simulink model "MotGenEvDynamic"  (R2022b)
settings: Solver=ode1  StartTime=0.0  StopTime=inf  FixedStep=TsElecDrive  RelTol=1e-3  EnableMultiTasking=on
model workspace (MAT data in the model file):
  EV_current = 200
  EV_motion = [20 4 0.8]
  EV_sf = 2000
  Fs = 0
  Fv = 0.0025
  Jcomp = 0.0227
  Ki = 25.1327
  Kisa = 346.6583
  Kp_d = 0.077049
  Kp_q = 0.1541
  Ksa = 85.4316
  Ksf = 1996.2651
  Ld = 6.13138564528e-05
  Ldq = [0.00075852 0.00084286]
  Lq = 0.000122627712906
  Mechanical = [0.0227 0.0025 0]
  P = 4
  PolePairs = 4
  Rs = 0.02
  T_max = 450
  T_mtpa = [0 42.1986572825 85.2083176897 129.729081531 176.299639273 225.306651971 277.019503371 331.625177598 389.25482581 450.002001304]
  ba = 3.4029
  id_mtpa = [0 -7.80314458768 -30.092823648 -64.186681647 -107.097717515 -156.321290228 -210.017144052 -266.906008079 -326.111998186 -387.032483343]
  idq0 = [0 0]
  idq_limits = [-387.027355555 779.385063397 870.190353311]
  iq_mtpa = [0 96.3724280977 191.019783835 282.872542968 371.626993516 457.46803527 540.777238675 621.964104296 701.396562769 779.382517017]
  lambda_pm = 0.0725
  mechanical = [0.0227 0.0025 0]
  omega_init = 0
  theta_init = 0
undefined symbols (not defined in the file): IO334, J, T_cpu, Tcpu, TsEV
libraries: speedgoatlib_hdlCoder_IO3xx x24, autolibmotorctrlr x1, HDL_Motor_Lib x1
settings Model: ModifiedByFormat=The MathWorks, Inc.  PauseTimes=10  Creator=The MathWorks, Inc.  LastModifiedBy=The MathWorks, Inc.
settings SolverCC: ConcurrentTasks=on  AlgebraicLoopSolver=TrustRegion  PositivePriorityOrder=on  AutoInsertRateTranBlk=on  DecoupledContinuousIntegration=on  MaxZcPerStep=1
settings DataIOCC: DSMLogging=off  ReturnWorkspaceOutputs=off
settings OptimizationCC: BlockReduction=off  UseFloatMulNetSlope=on  OptimizeBlockIOStorage=off
settings DebuggingCC: UnderspecifiedInitializationDetection=Classic  MergeDetectMultiDrivingBlocksExec=none  TasksWithSamePriorityMsg=none  UnconnectedInputMsg=warning  UnconnectedOutputMsg=warning  UnconnectedLineMsg=warning  SFMachineParentedDataDiag=warning  ArithmeticOperatorsInVariantConditions=warning
settings HardwareCC: ProdBitPerLong=64  ProdLongLongMode=on  ProdHWDeviceType=Intel->x86-64 (Linux 64)
settings ModelReferenceCC: EnableRefExpFcnMdlSchedulingChecks=on  PropagateSignalLabelsOutOfModel=off
settings SFSimCC: SimUseLocalCustomCode=off  MATLABDynamicMemAlloc=off  CustomCodeUndefinedFunction=UseInterfaceOnly
settings RTWCC: Description=Simulink Real-Time  SystemTargetFile=slrealtime.tlc  TemplateMakefile=slrealtime_default_tmf  RTWUseLocalCustomCode=off  Toolchain=Simulink Real-Time Toolchain  BuildConfiguration=Faster Runs  CodeExecutionProfiling=on  TargetLang=C++  DLArmComputeVersion=19.05
settings CodeAppCC: StateflowObjectComments=on
settings ConfigComp: CovMetricSettings=dsw  CovSaveCumulativeToWorkspaceVar=on  CovSaveSingleToWorkspaceVar=on  CovExternalEMLEnable=off
settings SimscapeCC: SimscapeNormalizeSystem=off

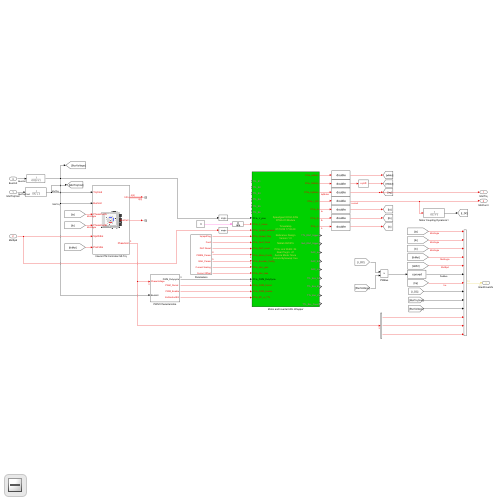
[thumbnail: Simulink's stored preview of the top-level diagram]
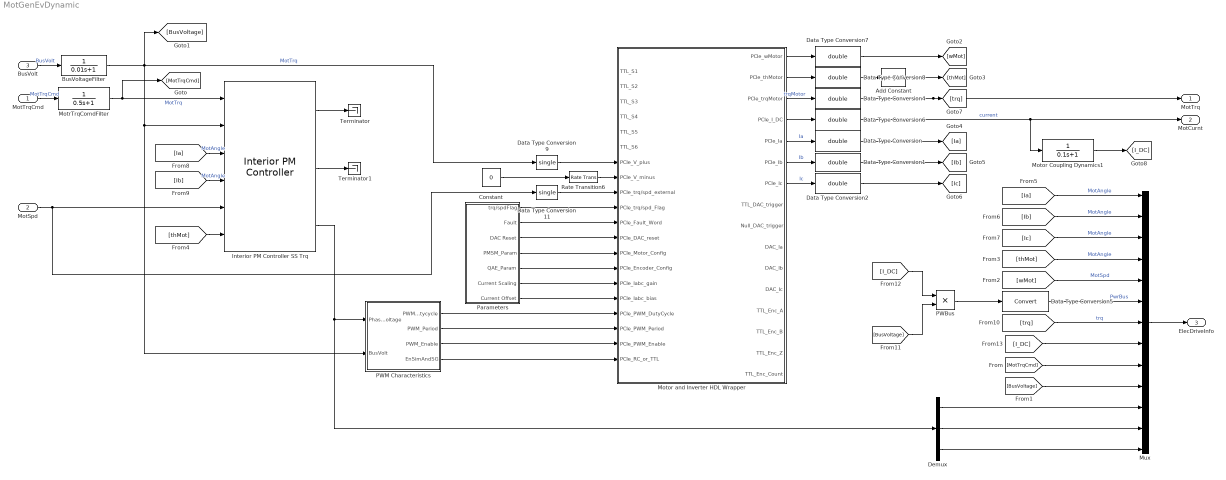
== system MotGenEvDynamic ==
  MotTrqCmd : Inport  OutDataTypeStr=double
  MotSpd : Inport  Port=2  OutDataTypeStr=double
  BusVolt : Inport  Port=3  OutDataTypeStr=double
  Add Constant : Bias  Bias=-pi/8  SaturateOnIntegerOverflow=off
  BusVoltageFilter : TransferFcn  Denominator=[0.01 1]
  Constant : Constant  Value=0  OutDataTypeStr=single
  Data Type Conversion{,1..2,4,6..8} (7 alike) : DataTypeConversion  OutDataTypeStr=double  SaturateOnIntegerOverflow=off  RndMeth=Floor
  Data Type Conversion11 : DataTypeConversion  OutDataTypeStr=single  SaturateOnIntegerOverflow=off  RndMeth=Floor
  Data Type Conversion5 : DataTypeConversion  SaturateOnIntegerOverflow=off  RndMeth=Floor
  Data Type Conversion9 : DataTypeConversion  OutDataTypeStr=single  SaturateOnIntegerOverflow=off  RndMeth=Floor
  Demux : Demux  Outputs=3
  Interior PM Controller SS Trq : autolibmotorctrlr/Interior PM Controller  control_type=Torque Control  Rs=Rs  Ld=Ld  Lq=Lq  lambda_pm=lambda_pm  PolePairs=PolePairs  Mechanical=Mechanical  MotorConstraint=Maximum Torque  T_max=T_max  I_max=44  bp=10  T_mtpa=T_mtpa  id_mtpa=id_mtpa  iq_mtpa=iq_mtpa  idq_limits=idq_limits  EV_current=EV_current  Tst=TsElecDrive  Kp_d=Kp_d  Kp_q=Kp_q  Ki=Ki/10  EV_motion=EV_motion  EV_sf=EV_sf  ba=ba  Ksa=Ksa  Kisa=Kisa  Ksf=Ksf  Jcomp=Jcomp  Fv=Fv  Fs=Fs  param_loss=Single efficiency measurement  eff=98  w_loss_bp=[0 200 400 600 800 1000]  T_loss_bp=[0 25 50 75 100]  losses_table=[100 100 100 100 100;100 150 200 250 300;100 200 300 400 500;100 250 400 550 700;100 300 500 700 900;100 350 600 850 1100]  w_eff_bp=[200 400 600 800 1000]  T_eff_bp=[25 50 75 100]  efficiency_table=[96.2 98.1 98.7 99;98.1 99 99.4 99.5;98.7 99.4 99.6 99.7;99 99.5 99.7 99.8;99.2 99.6 99.7 99.8]  x_w_bp=[-1000 -800 -600 -400 -200 200 400 600 800 1000]  x_T_bp=[-100 -75 -50 -25 25 50 75 100]  x_losses_mat=[200.400801603196 225.67703109328 200.803212851408 201.612903225806 199.999999999997 200 225 200;160.320641282556 180.541624874624 201.005025125625 202.020202020203 200 200 180 160;180.541624874624 180.722891566267 181.086519114686 197.568389057748 194.999999999999 179.999999999997 180 180;201.005025125625 181.086519114686 202.020202020203 193.67991845056 190 200 179.999999999997 200;202.020202020203 197.568389057748 193.67991845056 197.505197505197 190 190 194.999999999999 200;200 194.999999999999 190 190 197.505197505197 193.67991845056 197.568389057748 202.020202020203;200 179.999999999997 200 190 193.67991845056 202.020202020203 181.086519114686 201.005025125625;180 180 179.999999999997 194.999999999999 197.568389057748 181.086519114686 180.722891566267 180.541624874624;160 180 200 200 202.020202020203 201.005025125625 180.541624874624 160.320641282556;200 225 200 199.999999999997 201.612903225806 200.803212851408 225.67703109328 200.400801603196]  Tsm=5e-4
  Motor Coupling Dynamics1 : TransferFcn  Denominator=[0.1 1]
  Motor and Inverter HDL Wrapper : Subsystem  mask(Speedgoat IO334-325k Interface Block){module_id=1, slot=-1, ts=TsEV, OutputRange=Auto (same as ADC), PullRPort0=pull-down, VioPort0=3.3V, PullRPort1=pull-down, VioPort1=3.3V, PullRPort2=pull-down, VioPort2=3.3V, PullRPort3=pull-down, VioPort3=3.3V, PullRPort4=pull-down, VioPort4=3.3V, PullRPort5=pull-down, VioPort5=3.3V, PullRPort6=pull-down, VioPort6=3.3V, FpgaFreq=200}
      mask prompts: module_id "FPGA Module Identifier:"; slot "PCI slot (-1: autosearch):"; ts "Sample time:"; OutputRange "DAC Voltage Range:"; PullRPort0 "pull resistor"; VioPort0 "I/O voltage"; PullRPort1 "pull resistor"; VioPort1 "I/O voltage"; PullRPort2 "pull resistor"; VioPort2 "I/O voltage"; PullRPort3 "pull resistor"; VioPort3 "I/O voltage"; PullRPort4 "pull resistor"; VioPort4 "I/O voltage"; PullRPort5 "pull resistor"; VioPort5 "I/O voltage"; PullRPort6 "pull resistor"; VioPort6 "I/O voltage"; FpgaFreq "FPGA Frequency [MHz]"
      mask help: Simulink Real-Time Interface Block for Speedgoat IO334-325k.
      mask init:
      | hdlslrt.backend.mfpgaparameters;
      mask Help: eval('speedgoatdoc_hdlc')
      mask TypeOptions OutputRange: IO334 DAC Setup/OutputRange
      mask TypeOptions PullRPort0: Port Settings -2x/PullRPort0
      mask Callback PullRPort0: sg_fpga_HDLCoder_io3xx_2x_m(2)
      mask TypeOptions VioPort0: Port Settings -2x/VioPort0
      mask Callback VioPort0: sg_fpga_HDLCoder_io3xx_2x_m(2)
      mask TypeOptions PullRPort1: Port Settings -2x/PullRPort1
      mask Callback PullRPort1: sg_fpga_HDLCoder_io3xx_2x_m(2)
      mask TypeOptions VioPort1: Port Settings -2x/VioPort1
      mask Callback VioPort1: sg_fpga_HDLCoder_io3xx_2x_m(2)
      mask TypeOptions PullRPort2: Port Settings -2x/PullRPort2
      mask Callback PullRPort2: sg_fpga_HDLCoder_io3xx_2x_m(2)
      mask TypeOptions VioPort2: Port Settings -2x/VioPort2
      mask Callback VioPort2: sg_fpga_HDLCoder_io3xx_2x_m(2)
      mask TypeOptions PullRPort3: Port Settings -2x/PullRPort3
      mask Callback PullRPort3: sg_fpga_HDLCoder_io3xx_2x_m(2)
      mask TypeOptions VioPort3: Port Settings -2x/VioPort3
      mask Callback VioPort3: sg_fpga_HDLCoder_io3xx_2x_m(2)
      mask TypeOptions PullRPort4: Port Settings -2x/PullRPort4
      mask Callback PullRPort4: sg_fpga_HDLCoder_io3xx_2x_m(2)
      mask TypeOptions VioPort4: Port Settings -2x/VioPort4
      mask Callback VioPort4: sg_fpga_HDLCoder_io3xx_2x_m(2)
      mask TypeOptions PullRPort5: Port Settings -2x/PullRPort5
      mask Callback PullRPort5: sg_fpga_HDLCoder_io3xx_2x_m(2)
      mask TypeOptions VioPort5: Port Settings -2x/VioPort5
      mask Callback VioPort5: sg_fpga_HDLCoder_io3xx_2x_m(2)
      mask TypeOptions PullRPort6: Port Settings -2x/PullRPort6
      mask Callback PullRPort6: sg_fpga_HDLCoder_io3xx_2x_m(2)
      mask TypeOptions VioPort6: Port Settings -2x/VioPort6
      mask Callback VioPort6: sg_fpga_HDLCoder_io3xx_2x_m(2)
      mask DialogControl AnalogOutput Prompt: Analog Output
      mask DialogControl IO33421 Prompt: IO334-21
      mask DialogControl port1 Prompt: Port 1
      mask DialogControl port2 Prompt: Port 2
      mask DialogControl port3 Prompt: Port 3
      mask DialogControl port4 Prompt: Port 4
      mask DialogControl port5 Prompt: Port 5
      mask DialogControl port6 Prompt: Port 6
      mask DialogControl port7 Prompt: Port 7
      mask Display:
      | SetupBlkPath = find_system(gcb, 'LookUnderMasks', 'all', 'FollowLinks', 'on', 'regexp', 'on', 'Name', 'IO3(\d|x){2}\s+Setup' );
      | SetupBlkPath = SetupBlkPath{1};
      | TS = get_param(SetupBlkPath,'timestamp_mcs');
      | disp(sprintf('Speedgoat IO334-325k\nFPGA I/O Module\n\nTimestamp\n%s\n\nReference Design\nVersion 1.0\n\nMatlab R2021b\n\nPCIe Link Width: X4\nRear Plugin: -21\nAurora Mode: None\nAurora Byteswap: true\n', TS))
  MotrTrqComdFilter : TransferFcn  Denominator=[0.5 1]
  Mux : Mux  Inputs=13
  PWBus : Product
  PWM Characteristics : Subsystem
  Parameters : Subsystem
  Rate Transition6 : RateTransition
  Terminator : Terminator
  Terminator1 : Terminator
  MotTrq : Outport  VectorParamsAs1DForOutWhenUnconnected=off
  MotCurnt : Outport  Port=2  VectorParamsAs1DForOutWhenUnconnected=off
  ElecDriveInfo : Outport  Port=3  OutDataTypeStr=double  VectorParamsAs1DForOutWhenUnconnected=off
  wires:
  BusVolt/1 -> BusVoltageFilter/1  "BusVolt"
  MotSpd/1 -> Interior PM Controller SS Trq/5, Data Type Conversion11/1
  Interior PM Controller SS Trq/2 -> Terminator1/1
  Interior PM Controller SS Trq/1 -> Terminator/1
  Mux/1 -> ElecDriveInfo/1
  Demux/1 -> Mux/11
  Demux/2 -> Mux/12
  Demux/3 -> Mux/13
  Constant/1 -> Rate Transition6/1
  Parameters/7(Current Offset) -> Motor and Inverter HDL Wrapper/16(PCIe_Iabc_bias)
  Motor and Inverter HDL Wrapper/3(PCIe_trqMotor) -> Data Type Conversion4/1  "trqMotor"
  Motor and Inverter HDL Wrapper/2(PCIe_thMotor) -> Data Type Conversion8/1
  Motor and Inverter HDL Wrapper/4(PCIe_I_DC) -> Data Type Conversion6/1
  MotTrqCmd/1 -> MotrTrqComdFilter/1  "MotTrqCmd"
  PWBus/1 -> Data Type Conversion5/1
  Parameters/1(trq/spdFlag) -> Motor and Inverter HDL Wrapper/10(PCIe_trq/spd_Flag)
  Data Type Conversion11/1 -> Motor and Inverter HDL Wrapper/9(PCIe_trq/spd_external)
  Rate Transition6/1 -> Motor and Inverter HDL Wrapper/8(PCIe_V_minus)
  Parameters/4(PMSM_Param) -> Motor and Inverter HDL Wrapper/13(PCIe_Motor_Config)
  Parameters/5(QAE_Param) -> Motor and Inverter HDL Wrapper/14(PCIe_Encoder_Config)
  [trq] -> Mux/7  "trq"
  Data Type Conversion5/1 -> Mux/6  "PwrBus"
  Motor and Inverter HDL Wrapper/5(PCIe_Ia) -> Data Type Conversion/1  "Ia"
  Motor and Inverter HDL Wrapper/6(PCIe_Ib) -> Data Type Conversion1/1  "Ib"
  Motor and Inverter HDL Wrapper/7(PCIe_Ic) -> Data Type Conversion2/1  "Ic"
  Data Type Conversion9/1 -> Motor and Inverter HDL Wrapper/7(PCIe_V_plus)
  PWM Characteristics/4(EnSimAndSG) -> Motor and Inverter HDL Wrapper/20(PCIe_RC_or_TTL)
  Data Type Conversion4/1 -> [trq], MotTrq/1
  Parameters/2(Fault) -> Motor and Inverter HDL Wrapper/11(PCIe_Fault_Word)
  [wMot] -> Mux/5  "MotSpd"
  Interior PM Controller SS Trq/3 -> PWM Characteristics/1(PhaseVoltage), Demux/1
  [MotTrqCmd] -> Mux/9
  [BusVoltage] -> Mux/10
  PWM Characteristics/1(PWM_Dutycycle) -> Motor and Inverter HDL Wrapper/17(PCIe_PWM_DutyCycle)
  PWM Characteristics/2("PWM_Period ") -> Motor and Inverter HDL Wrapper/18(PCIe_PWM_Period)
  PWM Characteristics/3(PWM_Enable) -> Motor and Inverter HDL Wrapper/19(PCIe_PWM_Enable)
  Parameters/3(DAC Reset) -> Motor and Inverter HDL Wrapper/12(PCIe_DAC_reset)
  Motor and Inverter HDL Wrapper/1(PCIe_wMotor) -> Data Type Conversion7/1
  Data Type Conversion7/1 -> [wMot]
  Add Constant/1 -> [thMot]
  [thMot] -> Mux/4  "MotAngle"
  Data Type Conversion8/1 -> Add Constant/1
  [thMot] -> Interior PM Controller SS Trq/6
  Data Type Conversion/1 -> [Ia]
  Data Type Conversion1/1 -> [Ib]
  Data Type Conversion2/1 -> [Ic]
  [Ib] -> Mux/2  "MotAngle"
  [Ia] -> Mux/1  "MotAngle"
  [Ic] -> Mux/3  "MotAngle"
  [Ia] -> Interior PM Controller SS Trq/3  "MotAngle"
  [Ib] -> Interior PM Controller SS Trq/4  "MotAngle"
  Data Type Conversion6/1 -> Motor Coupling Dynamics1/1, MotCurnt/1  "current"
  [BusVoltage] -> PWBus/2
  Motor Coupling Dynamics1/1 -> [I_DC]
  [I_DC] -> PWBus/1
  [I_DC] -> Mux/8
  Parameters/6(Current Scaling) -> Motor and Inverter HDL Wrapper/15(PCIe_Iabc_gain)
  MotrTrqComdFilter/1 -> Interior PM Controller SS Trq/1, [MotTrqCmd]  "MotTrq"
  BusVoltageFilter/1 -> PWM Characteristics/2(BusVolt), Interior PM Controller SS Trq/2, [BusVoltage], Data Type Conversion9/1  "MotTrq"

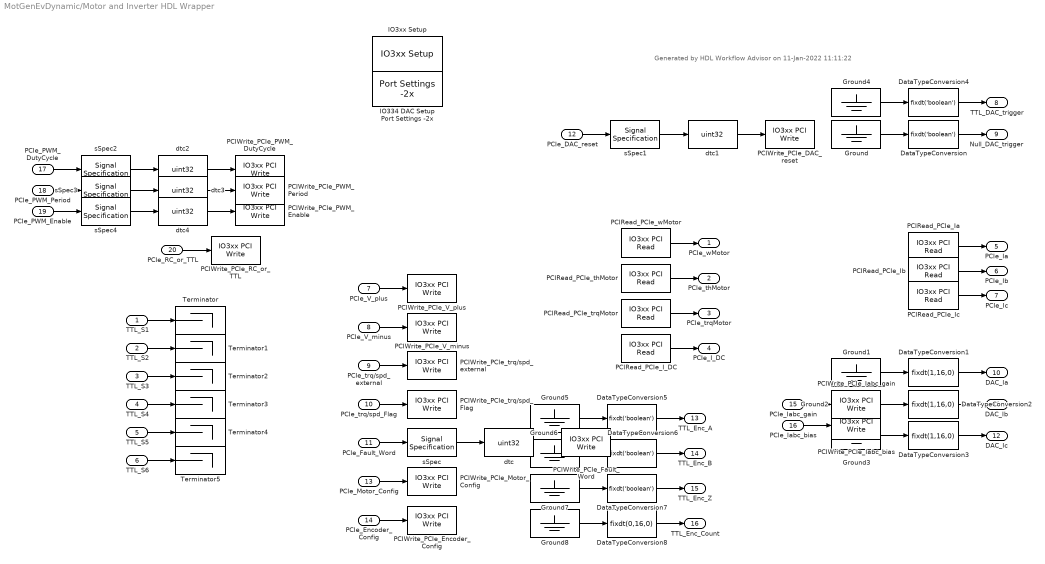
== system MotGenEvDynamic/Motor and Inverter HDL Wrapper ==
  note: Generated by HDL Workflow Advisor on 11-Jan-2022 11:11:22
  TTL_S1 : Inport
  TTL_S2 : Inport  Port=2
  TTL_S3 : Inport  Port=3
  TTL_S4 : Inport  Port=4
  TTL_S5 : Inport  Port=5
  TTL_S6 : Inport  Port=6
  PCIe_V_plus : Inport  Port=7
  PCIe_V_minus : Inport  Port=8
  PCIe_trq/spd_external : Inport  Port=9
  PCIe_trq/spd_Flag : Inport  Port=10
  PCIe_Fault_Word : Inport  Port=11
  PCIe_DAC_reset : Inport  Port=12
  PCIe_Motor_Config : Inport  Port=13
  PCIe_Encoder_Config : Inport  Port=14
  PCIe_Iabc_gain : Inport  Port=15
  PCIe_Iabc_bias : Inport  Port=16
  PCIe_PWM_DutyCycle : Inport  Port=17
  PCIe_PWM_Period : Inport  Port=18
  PCIe_PWM_Enable : Inport  Port=19
  PCIe_RC_or_TTL : Inport  Port=20
  DataTypeConversion{,4..7} (5 alike) : DataTypeConversion  OutDataTypeStr=fixdt('boolean')  ConvertRealWorld=Stored Integer (SI)  SaturateOnIntegerOverflow=off  RndMeth=Floor
  DataTypeConversion1 : DataTypeConversion  OutDataTypeStr=fixdt(1,16,0)  ConvertRealWorld=Stored Integer (SI)  SaturateOnIntegerOverflow=off  RndMeth=Floor
  DataTypeConversion2 : DataTypeConversion  OutDataTypeStr=fixdt(1,16,0)  ConvertRealWorld=Stored Integer (SI)  SaturateOnIntegerOverflow=off  RndMeth=Floor
  DataTypeConversion3 : DataTypeConversion  OutDataTypeStr=fixdt(1,16,0)  ConvertRealWorld=Stored Integer (SI)  SaturateOnIntegerOverflow=off  RndMeth=Floor
  DataTypeConversion8 : DataTypeConversion  OutDataTypeStr=fixdt(0,16,0)  ConvertRealWorld=Stored Integer (SI)  SaturateOnIntegerOverflow=off  RndMeth=Floor
  Ground{,1..8} (9 alike) : Ground
  IO334 DAC Setup : speedgoatlib_hdlCoder_IO3xx/IO334 DAC Setup  module_id=module_id  OutputRange=Auto (same as ADC)
  IO3xx Setup : speedgoatlib_hdlCoder_IO3xx/IO3xx Setup  mdl_ss_name=slrt_ex_pmsm/Motor and Inverter HDL Wrapper  board_type=IO334-325k  fpga_sync_mode=on  reset_mode=on  reset_mode_stop=off  device_id=1  module_id=module_id  pci_slot=slot  fpga_mat_file=hdl_prj\hdlsrc\slrt_ex_pmsm\MotorAndInverterHDLWrapper.mat  timestamp_mcs=01/10/22 17:02:49  timestamp=2201101544  tsreg=hex2dec('8')  bsf_file=MotorAndInverterHDLWrapperOriginal.mcs  mcs=0  init_reg_list=[]
  PCIRead_PCIe_I_DC : speedgoatlib_hdlCoder_IO3xx/IO3xx PCI Read  device_id=1  module_id=module_id  board_type=IO334-325k  port_name=PCIe_I_DC  port_offset=hex2dec('15C')  port_type=single  port_dim=1  strobe=0  sample_time=ts
  PCIRead_PCIe_Ia : speedgoatlib_hdlCoder_IO3xx/IO3xx PCI Read  device_id=1  module_id=module_id  board_type=IO334-325k  port_name=PCIe_Ia  port_offset=hex2dec('184')  port_type=single  port_dim=1  strobe=0  sample_time=ts
  PCIRead_PCIe_Ib : speedgoatlib_hdlCoder_IO3xx/IO3xx PCI Read  device_id=1  module_id=module_id  board_type=IO334-325k  port_name=PCIe_Ib  port_offset=hex2dec('188')  port_type=single  port_dim=1  strobe=0  sample_time=ts
  PCIRead_PCIe_Ic : speedgoatlib_hdlCoder_IO3xx/IO3xx PCI Read  device_id=1  module_id=module_id  board_type=IO334-325k  port_name=PCIe_Ic  port_offset=hex2dec('18C')  port_type=single  port_dim=1  strobe=0  sample_time=ts
  PCIRead_PCIe_thMotor : speedgoatlib_hdlCoder_IO3xx/IO3xx PCI Read  device_id=1  module_id=module_id  board_type=IO334-325k  port_name=PCIe_thMotor  port_offset=hex2dec('154')  port_type=single  port_dim=1  strobe=0  sample_time=ts
  PCIRead_PCIe_trqMotor : speedgoatlib_hdlCoder_IO3xx/IO3xx PCI Read  device_id=1  module_id=module_id  board_type=IO334-325k  port_name=PCIe_trqMotor  port_offset=hex2dec('158')  port_type=single  port_dim=1  strobe=0  sample_time=ts
  PCIRead_PCIe_wMotor : speedgoatlib_hdlCoder_IO3xx/IO3xx PCI Read  device_id=1  module_id=module_id  board_type=IO334-325k  port_name=PCIe_wMotor  port_offset=hex2dec('150')  port_type=single  port_dim=1  strobe=0  sample_time=ts
  PCIWrite_PCIe_DAC_reset : speedgoatlib_hdlCoder_IO3xx/IO3xx PCI Write  device_id=1  module_id=module_id  board_type=IO334-325k  port_name=PCIe_DAC_reset  port_offset=hex2dec('114')  port_type=uint32  port_dim=1  strobe=0  sample_time=ts
  PCIWrite_PCIe_Encoder_Config : speedgoatlib_hdlCoder_IO3xx/IO3xx PCI Write  device_id=1  module_id=module_id  board_type=IO334-325k  port_name=PCIe_Encoder_Config  port_offset=hex2dec('160')  port_type=single  port_dim=5  strobe=hex2dec('180')  sample_time=ts
  PCIWrite_PCIe_Fault_Word : speedgoatlib_hdlCoder_IO3xx/IO3xx PCI Write  device_id=1  module_id=module_id  board_type=IO334-325k  port_name=PCIe_Fault_Word  port_offset=hex2dec('110')  port_type=uint32  port_dim=1  strobe=0  sample_time=ts
  PCIWrite_PCIe_Iabc_bias : speedgoatlib_hdlCoder_IO3xx/IO3xx PCI Write  device_id=1  module_id=module_id  board_type=IO334-325k  port_name=PCIe_Iabc_bias  port_offset=hex2dec('11C')  port_type=single  port_dim=1  strobe=0  sample_time=ts
  PCIWrite_PCIe_Iabc_gain : speedgoatlib_hdlCoder_IO3xx/IO3xx PCI Write  device_id=1  module_id=module_id  board_type=IO334-325k  port_name=PCIe_Iabc_gain  port_offset=hex2dec('118')  port_type=single  port_dim=1  strobe=0  sample_time=ts
  PCIWrite_PCIe_Motor_Config : speedgoatlib_hdlCoder_IO3xx/IO3xx PCI Write  device_id=1  module_id=module_id  board_type=IO334-325k  port_name=PCIe_Motor_Config  port_offset=hex2dec('120')  port_type=single  port_dim=8  strobe=hex2dec('140')  sample_time=ts
  PCIWrite_PCIe_PWM_DutyCycle : speedgoatlib_hdlCoder_IO3xx/IO3xx PCI Write  device_id=1  module_id=module_id  board_type=IO334-325k  port_name=PCIe_PWM_DutyCycle  port_offset=hex2dec('190')  port_type=uint32  port_dim=3  strobe=hex2dec('1A0')  sample_time=ts
  PCIWrite_PCIe_PWM_Enable : speedgoatlib_hdlCoder_IO3xx/IO3xx PCI Write  device_id=1  module_id=module_id  board_type=IO334-325k  port_name=PCIe_PWM_Enable  port_offset=hex2dec('144')  port_type=uint32  port_dim=1  strobe=0  sample_time=ts
  PCIWrite_PCIe_PWM_Period : speedgoatlib_hdlCoder_IO3xx/IO3xx PCI Write  device_id=1  module_id=module_id  board_type=IO334-325k  port_name=PCIe_PWM_Period  port_offset=hex2dec('148')  port_type=uint32  port_dim=1  strobe=0  sample_time=ts
  PCIWrite_PCIe_RC_or_TTL : speedgoatlib_hdlCoder_IO3xx/IO3xx PCI Write  device_id=1  module_id=module_id  board_type=IO334-325k  port_name=PCIe_RC_or_TTL  port_offset=hex2dec('14C')  port_type=single  port_dim=1  strobe=0  sample_time=ts
  PCIWrite_PCIe_V_minus : speedgoatlib_hdlCoder_IO3xx/IO3xx PCI Write  device_id=1  module_id=module_id  board_type=IO334-325k  port_name=PCIe_V_minus  port_offset=hex2dec('104')  port_type=single  port_dim=1  strobe=0  sample_time=ts
  PCIWrite_PCIe_V_plus : speedgoatlib_hdlCoder_IO3xx/IO3xx PCI Write  device_id=1  module_id=module_id  board_type=IO334-325k  port_name=PCIe_V_plus  port_offset=hex2dec('100')  port_type=single  port_dim=1  strobe=0  sample_time=ts
  PCIWrite_PCIe_trq/spd_Flag : speedgoatlib_hdlCoder_IO3xx/IO3xx PCI Write  device_id=1  module_id=module_id  board_type=IO334-325k  port_name=PCIe_trq//spd_Flag  port_offset=hex2dec('10C')  port_type=single  port_dim=1  strobe=0  sample_time=ts
  PCIWrite_PCIe_trq/spd_external : speedgoatlib_hdlCoder_IO3xx/IO3xx PCI Write  device_id=1  module_id=module_id  board_type=IO334-325k  port_name=PCIe_trq//spd_external  port_offset=hex2dec('108')  port_type=single  port_dim=1  strobe=0  sample_time=ts
  Port Settings -2x : speedgoatlib_hdlCoder_IO3xx/Port Settings -2x  module_id=module_id  rearIO=-21  PullRPort0=pull-down  VioPort0=3.3V  PullRPort1=pull-down  VioPort1=3.3V  PullRPort2=pull-down  VioPort2=3.3V  PullRPort3=pull-down  VioPort3=3.3V  PullRPort4=pull-down  VioPort4=3.3V  PullRPort5=pull-down  VioPort5=3.3V  PullRPort6=pull-down  VioPort6=3.3V
  Terminator{,1..5} (6 alike) : Terminator
  dtc{,1..4} (5 alike) : DataTypeConversion  OutDataTypeStr=uint32  ConvertRealWorld=Stored Integer (SI)  SaturateOnIntegerOverflow=off
  sSpec : SignalSpecification  OutDataTypeStr=fixdt(0,32,0)
  sSpec1 : SignalSpecification  OutDataTypeStr=fixdt(0,16,0)
  sSpec2 : SignalSpecification  OutDataTypeStr=fixdt(0,32,0)
  sSpec3 : SignalSpecification  OutDataTypeStr=fixdt(0,32,0)
  sSpec4 : SignalSpecification  OutDataTypeStr=fixdt('boolean')
  PCIe_wMotor : Outport
  PCIe_thMotor : Outport  Port=2
  PCIe_trqMotor : Outport  Port=3
  PCIe_I_DC : Outport  Port=4
  PCIe_Ia : Outport  Port=5
  PCIe_Ib : Outport  Port=6
  PCIe_Ic : Outport  Port=7
  TTL_DAC_trigger : Outport  Port=8
  Null_DAC_trigger : Outport  Port=9
  DAC_Ia : Outport  Port=10
  DAC_Ib : Outport  Port=11
  DAC_Ic : Outport  Port=12
  TTL_Enc_A : Outport  Port=13
  TTL_Enc_B : Outport  Port=14
  TTL_Enc_Z : Outport  Port=15
  TTL_Enc_Count : Outport  Port=16
  wires:
  PCIe_V_plus/1 -> PCIWrite_PCIe_V_plus/1
  PCIe_V_minus/1 -> PCIWrite_PCIe_V_minus/1
  PCIe_trq/spd_external/1 -> PCIWrite_PCIe_trq/spd_external/1
  PCIe_trq/spd_Flag/1 -> PCIWrite_PCIe_trq/spd_Flag/1
  PCIe_Fault_Word/1 -> sSpec/1
  sSpec/1 -> dtc/1
  dtc/1 -> PCIWrite_PCIe_Fault_Word/1
  PCIe_DAC_reset/1 -> sSpec1/1
  sSpec1/1 -> dtc1/1
  dtc1/1 -> PCIWrite_PCIe_DAC_reset/1
  PCIe_Motor_Config/1 -> PCIWrite_PCIe_Motor_Config/1
  PCIe_Encoder_Config/1 -> PCIWrite_PCIe_Encoder_Config/1
  PCIe_Iabc_gain/1 -> PCIWrite_PCIe_Iabc_gain/1
  PCIe_Iabc_bias/1 -> PCIWrite_PCIe_Iabc_bias/1
  PCIe_PWM_DutyCycle/1 -> sSpec2/1
  sSpec2/1 -> dtc2/1
  dtc2/1 -> PCIWrite_PCIe_PWM_DutyCycle/1
  PCIe_PWM_Period/1 -> sSpec3/1
  sSpec3/1 -> dtc3/1
  dtc3/1 -> PCIWrite_PCIe_PWM_Period/1
  PCIe_PWM_Enable/1 -> sSpec4/1
  sSpec4/1 -> dtc4/1
  dtc4/1 -> PCIWrite_PCIe_PWM_Enable/1
  PCIe_RC_or_TTL/1 -> PCIWrite_PCIe_RC_or_TTL/1
  PCIRead_PCIe_wMotor/1 -> PCIe_wMotor/1
  PCIRead_PCIe_thMotor/1 -> PCIe_thMotor/1
  PCIRead_PCIe_trqMotor/1 -> PCIe_trqMotor/1
  PCIRead_PCIe_I_DC/1 -> PCIe_I_DC/1
  PCIRead_PCIe_Ia/1 -> PCIe_Ia/1
  PCIRead_PCIe_Ib/1 -> PCIe_Ib/1
  PCIRead_PCIe_Ic/1 -> PCIe_Ic/1
  DataTypeConversion/1 -> Null_DAC_trigger/1
  Ground/1 -> DataTypeConversion/1
  DataTypeConversion1/1 -> DAC_Ia/1
  Ground1/1 -> DataTypeConversion1/1
  DataTypeConversion2/1 -> DAC_Ib/1
  Ground2/1 -> DataTypeConversion2/1
  DataTypeConversion3/1 -> DAC_Ic/1
  Ground3/1 -> DataTypeConversion3/1
  TTL_S1/1 -> Terminator/1
  TTL_S2/1 -> Terminator1/1
  TTL_S3/1 -> Terminator2/1
  TTL_S4/1 -> Terminator3/1
  TTL_S5/1 -> Terminator4/1
  TTL_S6/1 -> Terminator5/1
  DataTypeConversion4/1 -> TTL_DAC_trigger/1
  Ground4/1 -> DataTypeConversion4/1
  DataTypeConversion5/1 -> TTL_Enc_A/1
  Ground5/1 -> DataTypeConversion5/1
  DataTypeConversion6/1 -> TTL_Enc_B/1
  Ground6/1 -> DataTypeConversion6/1
  DataTypeConversion7/1 -> TTL_Enc_Z/1
  Ground7/1 -> DataTypeConversion7/1
  DataTypeConversion8/1 -> TTL_Enc_Count/1
  Ground8/1 -> DataTypeConversion8/1

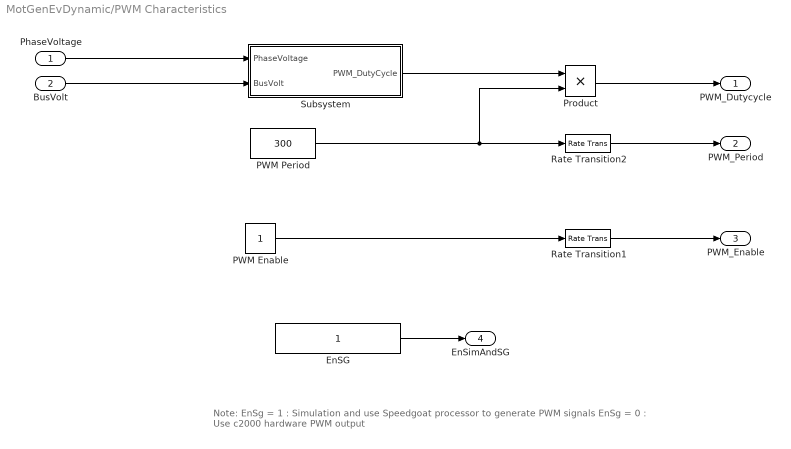
== system MotGenEvDynamic/PWM Characteristics ==
  note: Note:
      | EnSg = 1 : Simulation and use Speedgoat processor to generate PWM signals EnSg = 0 : Use c2000 hardware PWM output
  PhaseVoltage : Inport
  BusVolt : Inport  Port=2
  EnSG : Constant  OutDataTypeStr=single  SampleTime=-1
  PWM Enable : Constant  OutDataTypeStr=boolean
  PWM Period : Constant  Value=300  OutDataTypeStr=uint32
  Product : Product  OutDataTypeStr=uint32
  Rate Transition1 : RateTransition
  Rate Transition2 : RateTransition
  Subsystem : Subsystem
  PWM_Dutycycle : Outport
  "PWM_Period " : Outport  Port=2
  PWM_Enable : Outport  Port=3
  EnSimAndSG : Outport  Port=4
  wires:
  PWM Enable/1 -> Rate Transition1/1
  BusVolt/1 -> Subsystem/2(BusVolt)
  PWM Period/1 -> Product/2, Rate Transition2/1
  PhaseVoltage/1 -> Subsystem/1(PhaseVoltage)
  Subsystem/1(PWM_DutyCycle) -> Product/1
  Product/1 -> PWM_Dutycycle/1
  Rate Transition2/1 -> "PWM_Period "/1
  Rate Transition1/1 -> PWM_Enable/1
  EnSG/1 -> EnSimAndSG/1

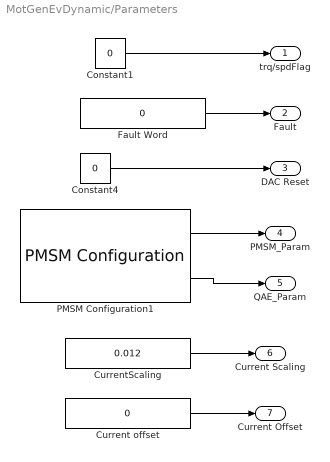
== system MotGenEvDynamic/Parameters ==
  Constant1 : Constant  Value=0  OutDataTypeStr=single  SampleTime=T_cpu
  Constant4 : Constant  Value=0  OutDataTypeStr=uint16  SampleTime=T_cpu
  Current offset : Constant  Value=0  OutDataTypeStr=single  SampleTime=-1
  CurrentScaling : Constant  Value=0.012  OutDataTypeStr=single  SampleTime=-1
  Fault Word : Constant  Value=0  OutDataTypeStr=uint32  SampleTime=T_cpu
  PMSM Configuration1 : HDL_Motor_Lib/PMSM Configuration  Ts=Tcpu  NPP=P  Lambda_pm=lambda_pm  Ld=Ld  Lq=Lq  Rs=Rs  J=J  numSlits=2000  shaftRotateDir=clockwise (CW)  shaftRotateDirIdx=1  zOffset=0  shaftInitialPos=0  zGateMode=pulse width = 180 el when channel A is high  zGateModeIdx=1
  trq/spdFlag : Outport
  Fault : Outport  Port=2
  DAC Reset : Outport  Port=3
  PMSM_Param : Outport  Port=4
  QAE_Param : Outport  Port=5
  Current Scaling : Outport  Port=6
  Current Offset : Outport  Port=7
  wires:
  Fault Word/1 -> Fault/1
  CurrentScaling/1 -> Current Scaling/1
  Current offset/1 -> Current Offset/1
  PMSM Configuration1/1 -> PMSM_Param/1
  PMSM Configuration1/2 -> QAE_Param/1
  Constant4/1 -> DAC Reset/1
  Constant1/1 -> trq/spdFlag/1

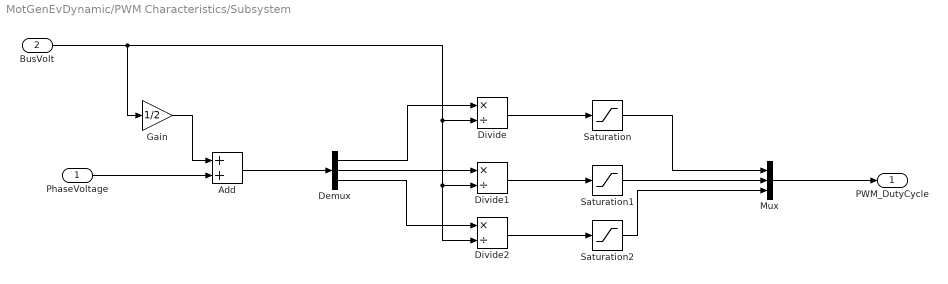
== system MotGenEvDynamic/PWM Characteristics/Subsystem ==
  PhaseVoltage : Inport
  BusVolt : Inport  Port=2
  Add : Sum
  Demux : Demux  Outputs=3
  Divide : Product  Inputs=*/
  Divide1 : Product  Inputs=*/
  Divide2 : Product  Inputs=*/
  Gain : Gain  Gain=1/2
  Mux : Mux  Inputs=3
  Saturation : Saturate  UpperLimit=1  LowerLimit=0
  Saturation1 : Saturate  UpperLimit=1  LowerLimit=0
  Saturation2 : Saturate  UpperLimit=1  LowerLimit=0
  PWM_DutyCycle : Outport
  wires:
  Mux/1 -> PWM_DutyCycle/1
  Demux/1 -> Divide/1
  BusVolt/1 -> Gain/1, Divide/2, Divide1/2, Divide2/2
  Demux/2 -> Divide1/1
  Demux/3 -> Divide2/1
  Divide/1 -> Saturation/1
  Divide1/1 -> Saturation1/1
  Divide2/1 -> Saturation2/1
  PhaseVoltage/1 -> Add/2
  Add/1 -> Demux/1
  Gain/1 -> Add/1
  Saturation/1 -> Mux/1
  Saturation1/1 -> Mux/2
  Saturation2/1 -> Mux/3
